simulink model "Env"  (R2020b)
settings: configuration reference "gen_config" (kept outside this file)
undefined symbols (not defined in the file): Drv_facSlopeWLTC_CUR, Drv_kmhDesWLTC_CUR, Env_facSlope, Env_kmhVehDes
settings Model: DataDictionary=Hybrid_vehicle.sldd  SimulationMode=accelerator  Creator=Georg  LastModifiedBy=jy
settings ConfigSetRef: SourceName=gen_config

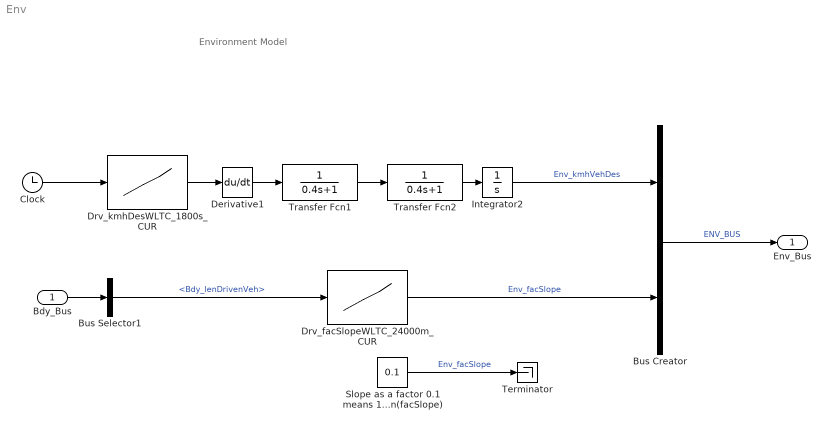
== system Env ==
  note: Environment Model
  Bdy_Bus : Inport  OutDataTypeStr=Bus: BDY_BUS
  Bus Creator : BusCreator  Inputs=Env_kmhVehDes,Env_facSlope  OutDataTypeStr=Bus: ENV_BUS  NonVirtualBus=on
  Bus Selector1 : BusSelector  OutputSignals=Bdy_lenDrivenVeh
  Clock : Clock
  Derivative1 : Derivative  CoefficientInTFapproximation=0.1
  Drv_facSlopeWLTC_24000m_CUR : Lookup  InputValues=Drv_facSlopeWLTC_CUR(:,1)  Table=Drv_facSlopeWLTC_CUR(:,2)  LookUpMeth=Interpolation-Use End Values
  Drv_kmhDesWLTC_1800s_CUR : Lookup  InputValues=Drv_kmhDesWLTC_CUR(:,1)  Table=Drv_kmhDesWLTC_CUR(:,2)  LookUpMeth=Interpolation-Use End Values
  Integrator2 : Integrator  UpperSaturationLimit=200.0001  LowerSaturationLimit=199.9999
  Slope as a factor 0.1 means 10 m climb on a basis of 100 m Angle alfa = arctan(facSlope) : Constant  Value=0.1
  Terminator : Terminator
  Transfer Fcn1 : TransferFcn  Denominator=[0.4 1]
  Transfer Fcn2 : TransferFcn  Denominator=[0.4 1]
  Env_Bus : Outport  OutDataTypeStr=Bus: ENV_BUS  VectorParamsAs1DForOutWhenUnconnected=off  BusOutputAsStruct=on
  wires:
  Transfer Fcn2/1 -> Integrator2/1
  Bdy_Bus/1 -> Bus Selector1/1
  Bus Selector1/1 -> Drv_facSlopeWLTC_24000m_CUR/1  "<Bdy_lenDrivenVeh>"
  Derivative1/1 -> Transfer Fcn1/1
  Drv_kmhDesWLTC_1800s_CUR/1 -> Derivative1/1
  Clock/1 -> Drv_kmhDesWLTC_1800s_CUR/1
  Integrator2/1 -> Bus Creator/1  "Env_kmhVehDes"
  Bus Creator/1 -> Env_Bus/1  "ENV_BUS"
  Transfer Fcn1/1 -> Transfer Fcn2/1
  Drv_facSlopeWLTC_24000m_CUR/1 -> Bus Creator/2  "Env_facSlope"
  Slope as a factor 0.1 means 10 m climb on a basis of 100 m Angle alfa = arctan(facSlope)/1 -> Terminator/1  "Env_facSlope"
